simulink model "task_6"  (R2023a)
settings: Solver=VariableStepAuto  StartTime=0.0  StopTime=1000  RelTol=1e-8
settings Model: Creator=user  LastModifiedBy=user

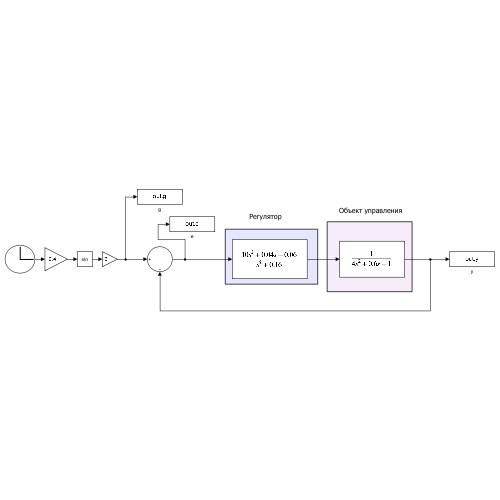
[thumbnail: Simulink's stored preview of the top-level diagram]
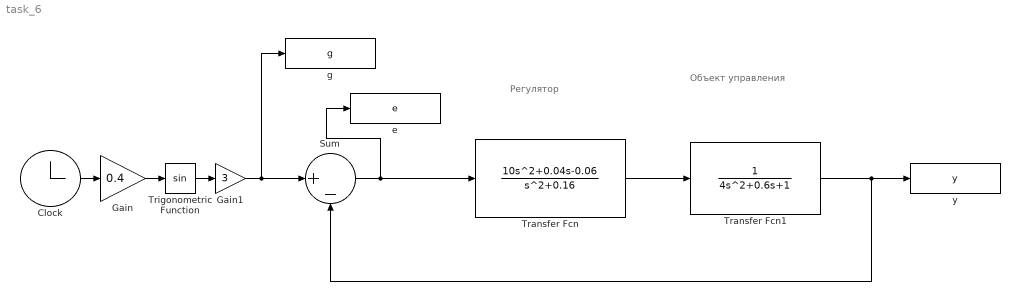
== system task_6 ==
  note: Объект управления
  note: Регулятор
  Clock : Clock
  Gain : Gain  Gain=0.4
  Gain1 : Gain  Gain=3
  Sum : Sum  Inputs=|+-
  Transfer Fcn : TransferFcn  Numerator=[10 0.04 -0.06]  Denominator=[1 0 0.16]
  Transfer Fcn1 : TransferFcn  Denominator=[4 0.6 1]
  Trigonometric Function : Trigonometry
  e : ToWorkspace  VariableName=e  SaveFormat=Timeseries  SampleTime=-1
  g : ToWorkspace  VariableName=g  SaveFormat=Timeseries  SampleTime=-1
  y : ToWorkspace  VariableName=y  SaveFormat=Timeseries  SampleTime=-1
  wires:
  Clock/1 -> Gain/1
  Gain/1 -> Trigonometric Function/1
  Trigonometric Function/1 -> Gain1/1
  Gain1/1 -> Sum/1, g/1
  Transfer Fcn1/1 -> Sum/2, y/1
  Sum/1 -> e/1, Transfer Fcn/1
  Transfer Fcn/1 -> Transfer Fcn1/1
